simulink model "PID"  (R2022a)
settings: Solver=FixedStepAuto  StartTime=0.0  StopTime=10.0  FixedStep=.01  RelTol=1e-3
settings Model: Creator=a2207206  LastModifiedBy=a2207206

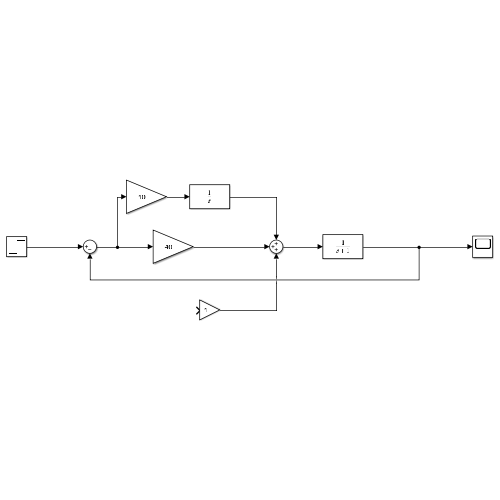
[thumbnail: Simulink's stored preview of the top-level diagram]
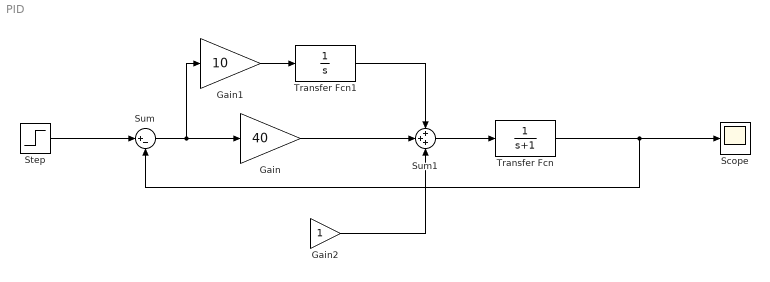
== system PID ==
  Gain : Gain  Gain=40
  Gain1 : Gain  Gain=10
  Gain2 : Gain
  Scope : Scope
  Step : Step  SampleTime=0
  Sum : Sum  Inputs=|+-
  Sum1 : Sum  Inputs=+++
  Transfer Fcn : TransferFcn  Denominator=[1 1]
  Transfer Fcn1 : TransferFcn  Denominator=[1 0]
  wires:
  Step/1 -> Sum/1
  Transfer Fcn/1 -> Sum/2, Scope/1
  Sum/1 -> Gain1/1, Gain/1
  Gain1/1 -> Transfer Fcn1/1
  Sum1/1 -> Transfer Fcn/1
  Transfer Fcn1/1 -> Sum1/1
  Gain/1 -> Sum1/2
  Gain2/1 -> Sum1/3
